simulink model "Test_Encoder_32_to_5"  (Simulink 8.7)
settings: Solver=ode45  StartTime=0.0  StopTime=len  RelTol=1e-3
libraries: Encoders_Lib x1, commutil2 x1, Miscellaneous x1
settings Model: Creator=N  LastModifiedBy=Jozko Mrkvicka
settings DataIOCC: LimitDataPoints=off
settings DebuggingCC: UnderspecifiedInitializationDetection=Simplified  MergeDetectMultiDrivingBlocksExec=error
settings HardwareCC: ProdBitPerPointer=64  ProdLargestAtomicFloat=Float  ProdIntDivRoundTo=Zero  ProdEndianess=LittleEndian  ProdHWDeviceType=Intel->x86-64 (Windows64)
settings ModelReferenceCC: PropagateSignalLabelsOutOfModel=on

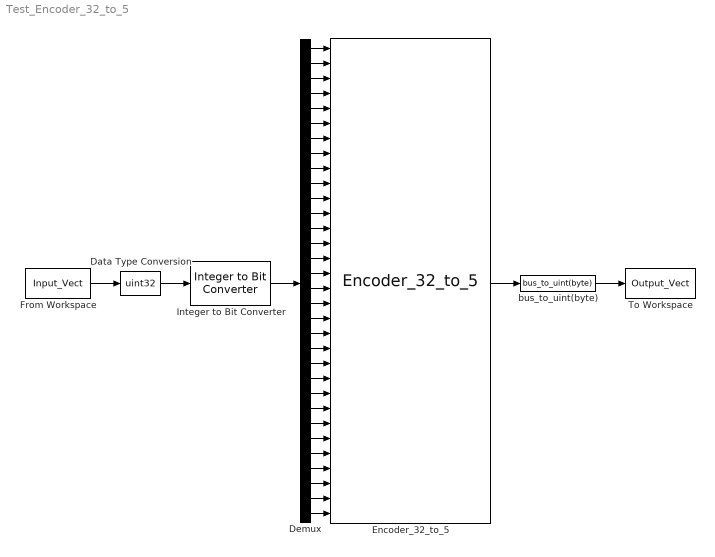
== system Test_Encoder_32_to_5 ==
  Data Type Conversion : DataTypeConversion  OutDataTypeStr=uint32
  Demux : Demux  Outputs=32
  Encoder_32_to_5 : Encoders_Lib/Encoders_Lib/Encoder_32_to_5
  From Workspace : FromWorkspace  VariableName=Input_Vect  SampleTime=1  Interpolate=off  OutputAfterFinalValue=Holding final value
  Integer to Bit Converter : commutil2/Integer to Bit Converter  nbits=32  signedInputValues=Unsigned  bitOrder=MSB first  outDtype=boolean
  To Workspace : ToWorkspace  VariableName=Output_Vect  SampleTime=1
  bus_to_uint(byte) : Miscellaneous/bus_to_uint(byte)
  wires:
  Encoder_32_to_5/1 -> bus_to_uint(byte)/1
  bus_to_uint(byte)/1 -> To Workspace/1
  Integer to Bit Converter/1 -> Demux/1
  Data Type Conversion/1 -> Integer to Bit Converter/1
  From Workspace/1 -> Data Type Conversion/1
  Demux/1 -> Encoder_32_to_5/1
  Demux/2 -> Encoder_32_to_5/2
  Demux/3 -> Encoder_32_to_5/3
  Demux/4 -> Encoder_32_to_5/4
  Demux/5 -> Encoder_32_to_5/5
  Demux/6 -> Encoder_32_to_5/6
  Demux/7 -> Encoder_32_to_5/7
  Demux/8 -> Encoder_32_to_5/8
  Demux/9 -> Encoder_32_to_5/9
  Demux/10 -> Encoder_32_to_5/10
  Demux/11 -> Encoder_32_to_5/11
  Demux/12 -> Encoder_32_to_5/12
  Demux/13 -> Encoder_32_to_5/13
  Demux/14 -> Encoder_32_to_5/14
  Demux/15 -> Encoder_32_to_5/15
  Demux/16 -> Encoder_32_to_5/16
  Demux/17 -> Encoder_32_to_5/17
  Demux/18 -> Encoder_32_to_5/18
  Demux/19 -> Encoder_32_to_5/19
  Demux/20 -> Encoder_32_to_5/20
  Demux/21 -> Encoder_32_to_5/21
  Demux/22 -> Encoder_32_to_5/22
  Demux/23 -> Encoder_32_to_5/23
  Demux/24 -> Encoder_32_to_5/24
  Demux/25 -> Encoder_32_to_5/25
  Demux/26 -> Encoder_32_to_5/26
  Demux/27 -> Encoder_32_to_5/27
  Demux/28 -> Encoder_32_to_5/28
  Demux/29 -> Encoder_32_to_5/29
  Demux/30 -> Encoder_32_to_5/30
  Demux/31 -> Encoder_32_to_5/31
  Demux/32 -> Encoder_32_to_5/32
